simulink model "Jacobian"  (R2025a)
settings: Solver=ode4  StartTime=0.0  StopTime=inf  FixedStep=1/500  RelTol=1e-3  EnableMultiTasking=on
undefined symbols (not defined in the file): HIL, Host, qc_get_step_size
libraries: quarc_library x7
settings Model: ExtModeTrigDuration=10000  Creator=fvranes  LastModifiedBy=rdu
settings SolverCC: AlgebraicLoopSolver=TrustRegion  PositivePriorityOrder=on
settings DataIOCC: ReturnWorkspaceOutputs=off
settings DebuggingCC: UnconnectedInputMsg=warning  UnconnectedOutputMsg=warning  UnconnectedLineMsg=warning  ArithmeticOperatorsInVariantConditions=warning
settings ModelReferenceCC: EnableRefExpFcnMdlSchedulingChecks=on
settings SFSimCC: SimUseLocalCustomCode=off  CustomCodeUndefinedFunction=UseInterfaceOnly
settings RTWCC: SystemTargetFile=quarc_win64.tlc  RTWUseLocalCustomCode=off  Toolchain=QUARC win64 | nmake (64-bit Windows)  BuildConfiguration=Faster Runs  GPUComputeCapability=3.5  Description=QUARC Win64 Target Using Toolchain
settings CodeAppCC: StateflowObjectComments=on
settings STFCustomTargetCC: SystemTargetFile=quarc_win64.tlc  TargetLangStandard=C99 (ISO)  MultiwordLength=2048.0  DynamicStringBufferSize=256.0  ConcurrentExecutionCompliant=on  UseToolchainInfoCompliant=on
settings GRTTargetCC: ExtModeMexFile=quarc_comm  ParMdlRefBuildCompliant=off  CompOptLevelCompliant=off  CombineOutputUpdateFcns=off  MatFileLogging=off  CPPClassGenCompliant=off  GRTInterface=on
settings ConfigComp: CovMetricSettings=dswe

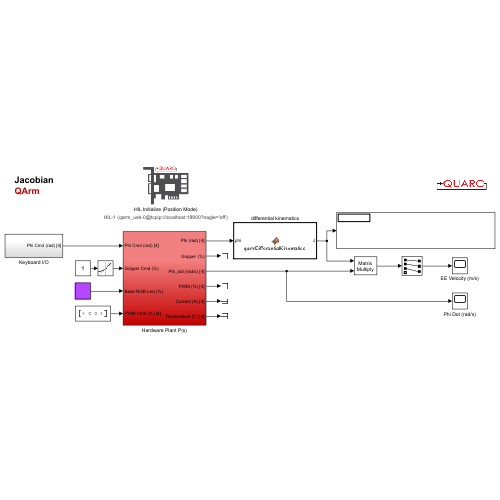
[thumbnail: Simulink's stored preview of the top-level diagram]
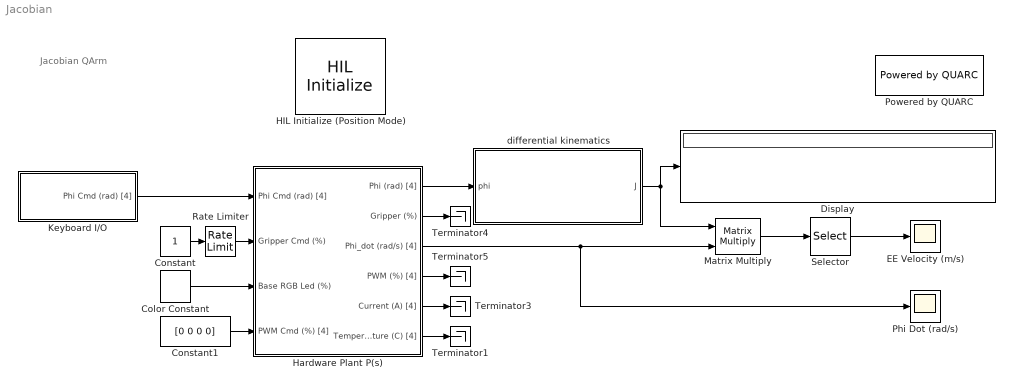
== system Jacobian ==
  note: Jacobian
      | QArm
  Color Constant : quarc_library/Sources/Signals/Color Constant  color=[0.71765 0.27451 1]
      settings: SourceProductName=QUARC Targets
  Constant : Constant
  Constant1 : Constant  Value=[0 0 0 0]
  Display : Display
      settings: Format=bank
  EE Velocity (m/s) : Scope
      settings: Title=End Effector Velocity (m/s)  ActiveDisplayYMinimum=-0.2  ActiveDisplayYMaximum=0.2  YLabel=m/s
  HIL Initialize (Position Mode) : quarc_library/Data Acquisition/Generic/Configuration/HIL Initialize  object_name=HIL-1  board_type=qarm_usb  board_number=0@tcpip://localhost:18900?nagle='off'  board_options=j0_mode=0;j1_mode=0;j2_mode=0;j3_mode=0;gripper_mode=0;  exclusive=off  active=on  hardware_clocks=[0]  clock_modes=[]  initial_clock_frequencies=[]  set_clock_params_at_start=off  set_clock_params_at_switch_in=off  set_clock_frequencies_at_start=off  set_clock_frequencies_at_switch_in=off  analog_input_channels=[5:9]  analog_input_configurations=[]  analog_input_maximums=[]  analog_input_minimums=[]  set_analog_input_params_at_start=off  set_analog_input_params_at_switch_in=off  analog_output_channels=[]  analog_output_maximums=inf  analog_output_minimums=-inf  initial_analog_outputs=[0]  final_analog_outputs=[0]  watchdog_analog_outputs=[]  set_analog_output_params_at_start=off  set_analog_output_params_at_switch_in=off  set_analog_outputs_at_start=off  set_analog_outputs_at_switch_in=off  set_analog_outputs_at_terminate=off  set_analog_outputs_at_switch_out=off  set_analog_outputs_on_watchdog=off  digital_input_channels=[]  digital_output_channels=[]  digital_output_configuration=[]  initial_digital_outputs=[0]  final_digital_outputs=[0]  watchdog_digital_outputs=[0]  set_digital_output_params_at_start=off  set_digital_output_params_at_switch_in=off  set_digital_outputs_at_start=off  set_digital_outputs_at_switch_in=off  set_digital_outputs_at_terminate=off  set_digital_outputs_at_switch_out=off  set_digital_outputs_on_watchdog=off  encoder_channels=[]  quadrature=[]  encoder_filter_frequency=[]  initial_encoder_counts=[]  set_encoder_params_at_start=off  set_encoder_params_at_switch_in=off  set_encoder_counts_at_start=off  set_encoder_counts_at_switch_in=off  pwm_channels=[]  pwm_modes=[]  pwm_frequency=[]  pwm_configuration=[]  pwm_alignment=[]  pwm_polarity=[]  pwm_leading_deadband=[]  pwm_trailing_deadband=[]  initial_pwm_outputs=[]  final_pwm_outputs=[]  watchdog_pwm_outputs=[]  set_pwm_params_at_start=off  set_pwm_params_at_switch_in=off  set_pwm_outputs_at_start=off  set_pwm_outputs_at_switch_in=off  set_pwm_outputs_at_terminate=off  set_pwm_outputs_at_switch_out=off  set_pwm_outputs_on_watchdog=off  other_output_channels=[1000:1004 11000:11003 11005:11007]  initial_other_outputs=[zeros(1,9), ones(1,3)]  final_other_outputs=[zeros(1,9), ones(1,3)]  watchdog_other_outputs=zeros(1,12)  set_other_outputs_at_start=off  set_other_outputs_at_switch_in=off  set_other_outputs_at_terminate=on  set_other_outputs_at_switch_out=off  set_other_outputs_on_watchdog=off
  Hardware Plant P(s) : Subsystem
  Keyboard I/O : Subsystem
  Matrix Multiply : Product  Multiplication=Matrix(*)
  Phi Dot (rad/s) : Scope
      settings: Title=Joint Velocities (rad/s)  ActiveDisplayYMinimum=-0.5  ActiveDisplayYMaximum=0.5  YLabel=rad/s
  Powered by QUARC : quarc_library/Logos/Powered by QUARC
  Rate Limiter : RateLimiter  SampleTimeMode=inherited
  Selector : Selector  InputPortWidth=4  IndexOptions=Index vector (dialog)  Indices=[1:3]  OutputSizes=1
  Terminator{1,3..5} (4 alike) : Terminator
  differential kinematics : MATLAB Function  TreatAsAtomicUnit=on
  wires:
  Color Constant/1 -> Hardware Plant P(s)/3(Base RGB Led (%))
  Constant1/1 -> Hardware Plant P(s)/4(PWM Cmd (%) [4])
  Hardware Plant P(s)/6(Temperature (C) [4]) -> Terminator1/1
  Hardware Plant P(s)/3(Phi_dot (rad/s) [4]) -> Phi Dot (rad/s)/1, Matrix Multiply/2
  Hardware Plant P(s)/5(Current (A) [4]) -> Terminator3/1
  Rate Limiter/1 -> Hardware Plant P(s)/2(Gripper Cmd (%))
  Hardware Plant P(s)/2(Gripper (%)) -> Terminator4/1
  Hardware Plant P(s)/4(PWM (%) [4]) -> Terminator5/1
  Keyboard I/O/1(Phi Cmd (rad) [4]) -> Hardware Plant P(s)/1(Phi Cmd (rad) [4])
  Constant/1 -> Rate Limiter/1
  differential kinematics/1(J) -> Matrix Multiply/1, Display/1
  Hardware Plant P(s)/1(Phi (rad) [4]) -> differential kinematics/1(phi)
  Matrix Multiply/1 -> Selector/1
  Selector/1 -> EE Velocity (m/s)/1

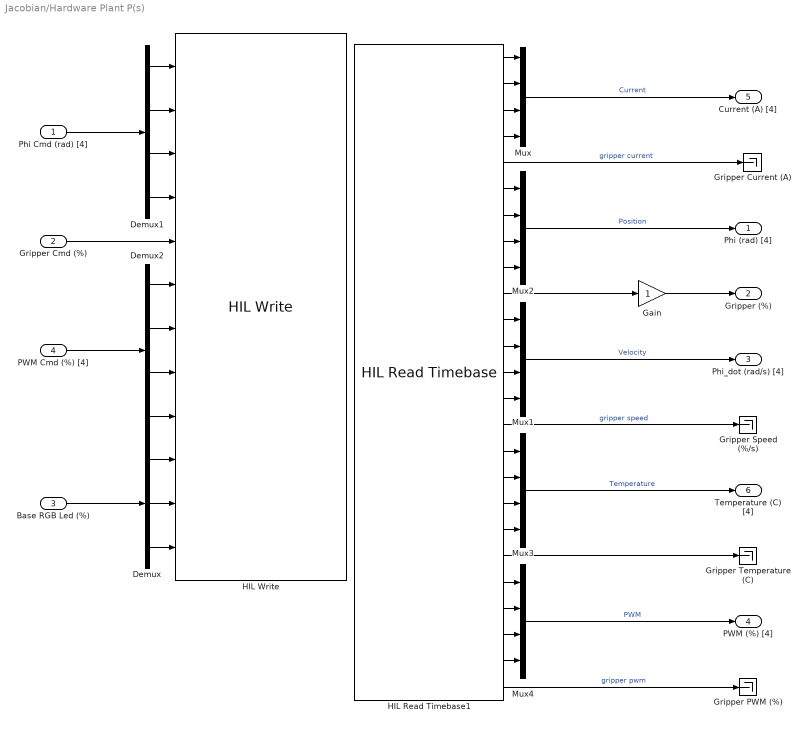
== system Jacobian/Hardware Plant P(s) ==
  Phi Cmd (rad) [4] : Inport
  Gripper Cmd (%) : Inport  Port=2
  Base RGB Led (%) : Inport  Port=3
  PWM Cmd (%) [4] : Inport  Port=4
  Demux : Demux  Outputs=3
  Demux1 : Demux
  Demux2 : Demux
  Gain : Gain
  Gripper Current (A) : Terminator
  Gripper PWM (%) : Terminator
  Gripper Speed (%/s) : Terminator
  Gripper Temperature (C) : Terminator
  HIL Read Timebase1 : quarc_library/Data Acquisition/Generic/Timebases/HIL Read Timebase  object_name=HIL-1  clock=0  analog_channels=[5:9]  encoder_channels=[]  digital_channels=[]  other_channels=[1000:1004 3000:3004 10000:10004 11000:11004]  active=on  vector_output=off  data_type_mode=Inherit via back propagation  encoder_data_type=double  digital_data_type=boolean  overflow_mode=Synchronize (for simulated cards only)  samples_in_buffer=1
  HIL Write : quarc_library/Data Acquisition/Generic/Immediate I//O/HIL Write  object_name=HIL-1  analog_channels=[]  pwm_channels=[]  digital_channels=[]  other_channels=[1000:1004 11000:11003 11005:11007]  sample_time=-1  active=on  vector_input=off
  Mux{,1..4} (5 alike) : Mux
  Phi (rad) [4] : Outport  VectorParamsAs1DForOutWhenUnconnected=off
  Gripper (%) : Outport  Port=2  VectorParamsAs1DForOutWhenUnconnected=off
  Phi_dot (rad/s) [4] : Outport  Port=3  VectorParamsAs1DForOutWhenUnconnected=off
  PWM (%) [4] : Outport  Port=4  VectorParamsAs1DForOutWhenUnconnected=off
  Current (A) [4] : Outport  Port=5  VectorParamsAs1DForOutWhenUnconnected=off
  Temperature (C) [4] : Outport  Port=6  VectorParamsAs1DForOutWhenUnconnected=off
  wires:
  HIL Read Timebase1/14 -> Mux1/4
  HIL Read Timebase1/9 -> Mux2/4
  HIL Read Timebase1/6 -> Mux2/1
  HIL Read Timebase1/18 -> Mux3/3
  HIL Read Timebase1/8 -> Mux2/3
  HIL Read Timebase1/12 -> Mux1/2
  HIL Read Timebase1/4 -> Mux/4
  HIL Read Timebase1/7 -> Mux2/2
  HIL Read Timebase1/5 -> Gripper Current (A)/1  "gripper current"
  HIL Read Timebase1/15 -> Gripper Speed (%/s)/1  "gripper speed"
  Demux/3 -> HIL Write/12
  HIL Read Timebase1/3 -> Mux/3
  HIL Read Timebase1/17 -> Mux3/2
  HIL Read Timebase1/16 -> Mux3/1
  HIL Read Timebase1/11 -> Mux1/1
  Demux/1 -> HIL Write/10
  HIL Read Timebase1/19 -> Mux3/4
  Demux/2 -> HIL Write/11
  HIL Read Timebase1/13 -> Mux1/3
  HIL Read Timebase1/2 -> Mux/2
  HIL Read Timebase1/1 -> Mux/1
  HIL Read Timebase1/20 -> Gripper Temperature (C)/1
  Mux/1 -> Current (A) [4]/1  "Current"
  Mux1/1 -> Phi_dot (rad/s) [4]/1  "Velocity"
  Mux3/1 -> Temperature (C) [4]/1  "Temperature"
  Base RGB Led (%)/1 -> Demux/1
  Demux1/1 -> HIL Write/1
  Demux1/2 -> HIL Write/2
  Demux1/3 -> HIL Write/3
  Demux1/4 -> HIL Write/4
  Phi Cmd (rad) [4]/1 -> Demux1/1
  PWM Cmd (%) [4]/1 -> Demux2/1
  Demux2/1 -> HIL Write/6
  Demux2/2 -> HIL Write/7
  Demux2/3 -> HIL Write/8
  Demux2/4 -> HIL Write/9
  Mux2/1 -> Phi (rad) [4]/1  "Position"
  HIL Read Timebase1/21 -> Mux4/1
  HIL Read Timebase1/22 -> Mux4/2
  HIL Read Timebase1/23 -> Mux4/3
  HIL Read Timebase1/24 -> Mux4/4
  HIL Read Timebase1/25 -> Gripper PWM (%)/1  "gripper pwm"
  Mux4/1 -> PWM (%) [4]/1  "PWM"
  HIL Read Timebase1/10 -> Gain/1
  Gain/1 -> Gripper (%)/1
  Gripper Cmd (%)/1 -> HIL Write/5

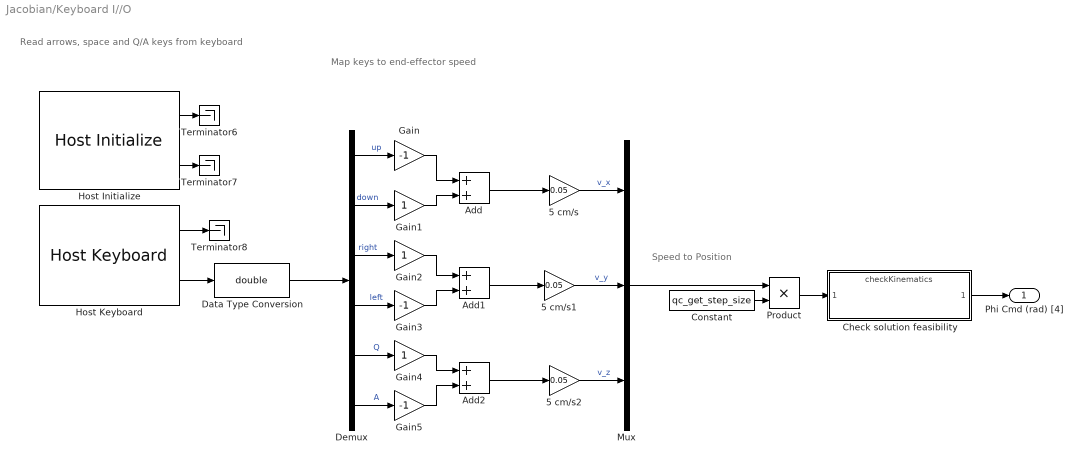
== system Jacobian/Keyboard I//O ==
  note: Map keys to end-effector speed
  note: Read arrows, space and Q/A keys
      | from keyboard
  note: Speed to Position
  5 cm/s : Gain  Gain=0.05
  5 cm/s1 : Gain  Gain=0.05
  5 cm/s2 : Gain  Gain=0.05
  Add : Sum
  Add1 : Sum
  Add2 : Sum
  Check solution feasibility : ModelReference  ModelNameDialog=checkKinematics.slxp  ModelReferenceVersion=1.13  CopyOfModelProtected=on
  Constant : Constant  Value=qc_get_step_size
  Data Type Conversion : DataTypeConversion  OutDataTypeStr=double  SaturateOnIntegerOverflow=off  RndMeth=Floor
  Demux : Demux  Outputs=6
  Gain : Gain  Gain=-1
  Gain1 : Gain
  Gain2 : Gain
  Gain3 : Gain  Gain=-1
  Gain4 : Gain
  Gain5 : Gain  Gain=-1
  Host Initialize : quarc_library/Devices/Peripherals/Host/Host Initialize  object_name=Host-1  uri_source=Use external mode communications  uri=tcpip://localhost:18001  send_buffer_size=1000  receive_buffer_size=1000  thread_priority=0  run_client=on  use_window=off  window_position=[]  sample_time=qc_get_step_size  active=on
      settings: SourceProductName=QUARC Targets
  Host Keyboard : quarc_library/Devices/Peripherals/Host/Host Keyboard  object_name=Host-1  virtual_key="[38  40  39  37  81  65]"  sample_time=qc_get_step_size  enabled=on  debug_mode=off
      settings: SourceProductName=QUARC Targets
  Mux : Mux  Inputs=3
  Product : Product
  Terminator6 : Terminator
  Terminator7 : Terminator
  Terminator8 : Terminator
  Phi Cmd (rad) [4] : Outport  VectorParamsAs1DForOutWhenUnconnected=off
  wires:
  Host Keyboard/1 -> Terminator8/1
  Host Initialize/2 -> Terminator7/1
  Host Initialize/1 -> Terminator6/1
  Host Keyboard/2 -> Data Type Conversion/1
  Data Type Conversion/1 -> Demux/1
  Check solution feasibility/1 -> Phi Cmd (rad) [4]/1
  Product/1 -> Check solution feasibility/1
  Mux/1 -> Product/1
  Constant/1 -> Product/2
  Demux/1 -> Gain/1  "up"
  Demux/2 -> Gain1/1  "down"
  Demux/3 -> Gain2/1  "right"
  Demux/4 -> Gain3/1  "left"
  Demux/5 -> Gain4/1  "Q"
  Demux/6 -> Gain5/1  "A"
  5 cm/s/1 -> Mux/1  "v_x"
  5 cm/s1/1 -> Mux/2  "v_y"
  5 cm/s2/1 -> Mux/3  "v_z"
  Gain1/1 -> Add/2
  Gain/1 -> Add/1
  Gain2/1 -> Add1/1
  Gain3/1 -> Add1/2
  Gain4/1 -> Add2/1
  Gain5/1 -> Add2/2
  Add/1 -> 5 cm/s/1
  Add1/1 -> 5 cm/s1/1
  Add2/1 -> 5 cm/s2/1

== matlab function Jacobian/differential kinematics ==
  data: phi input; J output
function J   = qarmDifferentialKinematics(phi)

%% QUANSER_ARM_FDK
% v 1.0 - 13th August 2020

% REFERENCE: 
% Chapter 5. Velocity Kinematics
% Robot Dynamics and Control 
% Spong, Vidyasagar
% 1989

% INPUTS:
% phi     : Alternate joint angles vector 4 x 1

% OUTPUTS:
% p4      : End-effector frame {4} position vector expressed in base frame {0}
% R04     : rotation matrix from end-effector frame {4} to base frame {0}

%% Manipulator parameters:
L1 = 0.1400;
L2 = 0.3500;
L3 = 0.0500;
L4 = 0.2500;
L5 = 0.1500;

%% Alternate parameters
l1 = L1;
l2 = sqrt(L2^2 + L3^2);
l3 = L4 + L5;
beta = atan(L3/L2);

%% From phi space to theta space 
theta = phi;
theta(1) = phi(1);
theta(2) = phi(2) + beta - pi/2;
theta(3) = phi(3) - beta;
theta(4) = phi(4);

%% Jacobian term definition:

J = eye(4);
J(1,1) = ; 
J(1,2) = ; 
J(1,3) = ; 
J(1,4) = ;
J(2,1) = ; 
J(2,2) = ;
J(2,3) = ;
J(2,4) = ;
J(3,1) = ;
J(3,2) = ;
J(3,3) = ;
J(3,4) = ;
J(4,1) = ;
J(4,2) = ;
J(4,3) = ;
J(4,4) = ;

end
